simulink model "untitled"  (R2024b)
settings: Solver=VariableStepAuto  StartTime=0.0  StopTime=15.0  RelTol=1e-3
settings Model: Creator=DT User  LastModifiedBy=DT User

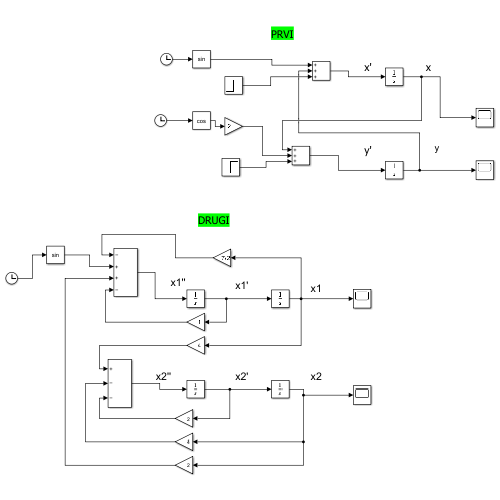
[thumbnail: Simulink's stored preview of the top-level diagram]
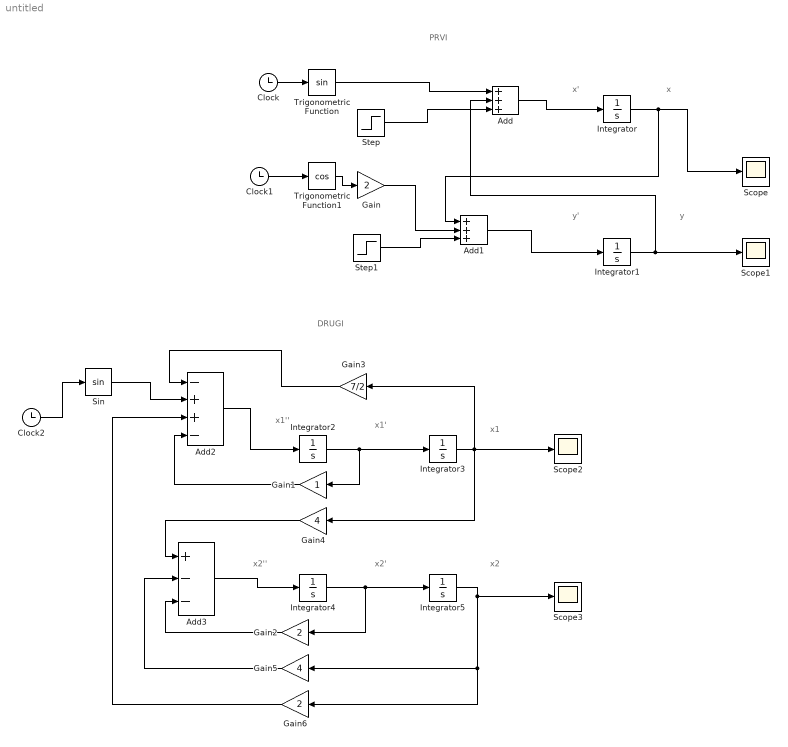
== system untitled ==
  note: DRUGI
  note: x1
  note: y'
  note: x'
  note: x
  note: y
  note: x1'
  note: x1''
  note: x2'
  note: x2
  note: x2''
  note: PRVI
  Add : Sum  Inputs=+++
  Add1 : Sum  Inputs=+++
  Add2 : Sum  Inputs=-++-
  Add3 : Sum  Inputs=+--
  Clock : Clock
  Clock1 : Clock
  Clock2 : Clock
  Gain : Gain  Gain=2
  Gain1 : Gain
  Gain2 : Gain  Gain=2
  Gain3 : Gain  Gain=7/2
  Gain4 : Gain  Gain=4
  Gain5 : Gain  Gain=4
  Gain6 : Gain  Gain=2
  Integrator : Integrator  InitialCondition=2
  Integrator{1..5} (5 alike) : Integrator
  Scope{,1..3} (4 alike) : Scope
  Sin : Trigonometry
  Step : Step  SampleTime=0
  Step1 : Step  SampleTime=0
  Trigonometric Function : Trigonometry
  Trigonometric Function1 : Trigonometry  Operator=cos
  wires:
  Clock/1 -> Trigonometric Function/1
  Trigonometric Function1/1 -> Gain/1
  Trigonometric Function/1 -> Add/1
  Add/1 -> Integrator/1
  Integrator/1 -> Add1/1, Scope/1
  Add1/1 -> Integrator1/1
  Integrator1/1 -> Add/2, Scope1/1
  Gain/1 -> Add1/2
  Clock1/1 -> Trigonometric Function1/1
  Step/1 -> Add/3
  Step1/1 -> Add1/3
  Integrator2/1 -> Gain1/1, Integrator3/1
  Integrator4/1 -> Gain2/1, Integrator5/1
  Clock2/1 -> Sin/1
  Sin/1 -> Add2/2
  Add2/1 -> Integrator2/1
  Gain1/1 -> Add2/4
  Gain3/1 -> Add2/1
  Integrator3/1 -> Gain4/1, Scope2/1, Gain3/1
  Gain4/1 -> Add3/1
  Gain2/1 -> Add3/3
  Add3/1 -> Integrator4/1
  Gain5/1 -> Add3/2
  Integrator5/1 -> Scope3/1, Gain6/1, Gain5/1
  Gain6/1 -> Add2/3
